simulink model "EPD629_WilliamsJ_AS09_Simulink"  (R2021b)
settings: Solver=VariableStepAuto  StartTime=0.0  StopTime=0.3  MaxStep=0.001  RelTol=1e-3
values from neighbouring files (symbols this model uses):
  b = .001    (= 0.001)    [EPD629_WilliamsJ_AS09.m]
  J = 50e-6    (= 5e-05)    [EPD629_WilliamsJ_AS09.m]
  K = 0.1    [EPD629_WilliamsJ_AS09.m]
  Kb = Kt    (= 0.063)    [EPD629_WilliamsJ_AS09.m]
  Kd5 = NUM{1}(1)    [EPD629_WilliamsJ_AS09.m]
  Ki1 = NUM{1}(2)    [EPD629_WilliamsJ_AS09.m]
  Ki2 = NUM{1}(2)    [EPD629_WilliamsJ_AS09.m]
  Ki3 = NUM{1}(2)    [EPD629_WilliamsJ_AS09.m]
  Ki4 = NUM{1}(2)    [EPD629_WilliamsJ_AS09.m]
  Ki5 = NUM{1}(3)    [EPD629_WilliamsJ_AS09.m]
  Kp1 = NUM{1}(1)    [EPD629_WilliamsJ_AS09.m]
  Kp2 = NUM{1}(1)    [EPD629_WilliamsJ_AS09.m]
  Kp3 = NUM{1}(1)    [EPD629_WilliamsJ_AS09.m]
  Kp4 = NUM{1}(1)    [EPD629_WilliamsJ_AS09.m]
  Kp5 = NUM{1}(2)    [EPD629_WilliamsJ_AS09.m]
  Kt = 0.063    [EPD629_WilliamsJ_AS09.m]
  L = 1e-4    (= 0.0001)    [EPD629_WilliamsJ_AS09.m]
  R = 0.35    [EPD629_WilliamsJ_AS09.m]
  Tau = 0.001    [EPD629_WilliamsJ_AS09.m]
settings Model: Creator=justin  LastModifiedBy=justin

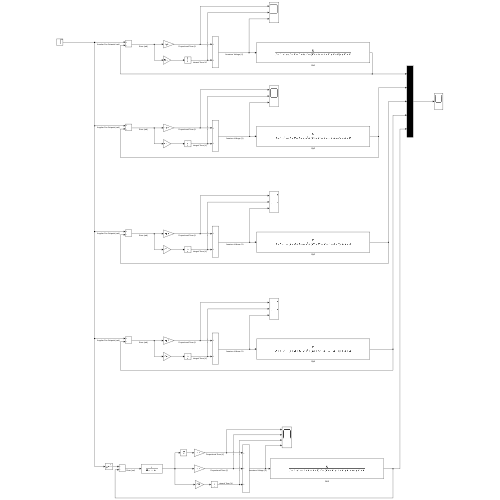
[thumbnail: Simulink's stored preview of the top-level diagram]
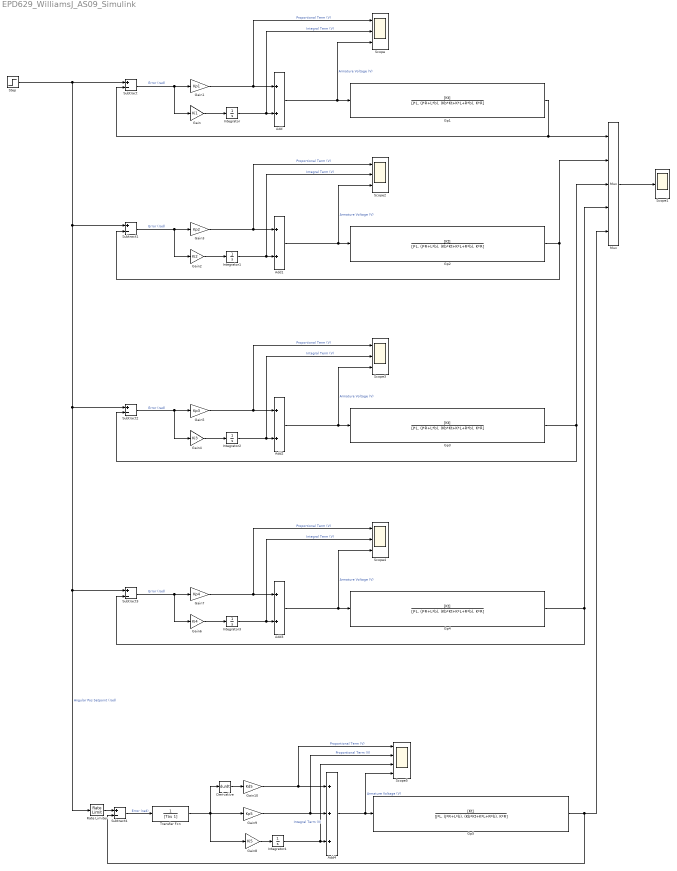
== system EPD629_WilliamsJ_AS09_Simulink ==
  Add{,1..3} (4 alike) : Sum
  Add4 : Sum  Inputs=+++
  Derivative : Derivative
  Gain : Gain  Gain=Ki1
  Gain1 : Gain  Gain=Kp1
  Gain10 : Gain  Gain=Kd5
  Gain2 : Gain  Gain=Ki2
  Gain3 : Gain  Gain=Kp2
  Gain4 : Gain  Gain=Ki3
  Gain5 : Gain  Gain=Kp3
  Gain6 : Gain  Gain=Ki4
  Gain7 : Gain  Gain=Kp4
  Gain8 : Gain  Gain=Ki5
  Gain9 : Gain  Gain=Kp5
  Gp{1..5} (5 alike) : TransferFcn  Numerator=[Kt]  Denominator=[J*L, (J*R+L*b), (Kb*Kt+K*L+R*b), K*R]
  Integrator{,1..4} (5 alike) : Integrator
  Mux : Mux  Inputs=5
  Rate Limiter : RateLimiter  RisingSlewLimit=180  FallingSlewLimit=-180  SampleTimeMode=inherited
  Scope{,2..4} (4 alike) : Scope  NumInputPorts=3
  Scope1 : Scope
  Scope5 : Scope  NumInputPorts=4
  Step : Step  Time=0.1  SampleTime=0
  Subtract{,1..4} (5 alike) : Sum  Inputs=+-
  Transfer Fcn : TransferFcn  Denominator=[Tau 1]
  wires:
  Subtract/1 -> Gain1/1, Gain/1  "Error (rad)"
  Gain/1 -> Integrator/1
  Gain1/1 -> Add/1, Scope/1  "Proportional Term (V)"
  Integrator/1 -> Add/2, Scope/2  "Integral Term (V)"
  Add/1 -> Gp1/1, Scope/3  "Armature Voltage (V)"
  Gp1/1 -> Subtract/2, Mux/1
  Mux/1 -> Scope1/1
  Gp2/1 -> Mux/2, Subtract1/2
  Add1/1 -> Gp2/1, Scope2/3  "Armature Voltage (V)"
  Integrator1/1 -> Scope2/2, Add1/2  "Integral Term (V)"
  Gain3/1 -> Scope2/1, Add1/1  "Proportional Term (V)"
  Gain2/1 -> Integrator1/1
  Subtract1/1 -> Gain2/1, Gain3/1  "Error (rad)"
  Subtract2/1 -> Gain5/1, Gain4/1  "Error (rad)"
  Gain4/1 -> Integrator2/1
  Gain5/1 -> Add2/1, Scope3/1  "Proportional Term (V)"
  Integrator2/1 -> Add2/2, Scope3/2  "Integral Term (V)"
  Add2/1 -> Scope3/3, Gp3/1  "Armature Voltage (V)"
  Gp3/1 -> Mux/3, Subtract2/2
  Step/1 -> Rate Limiter/1, Subtract3/1, Subtract2/1, Subtract1/1, Subtract/1  "Angular Pos Setpoint (rad)"
  Gp4/1 -> Subtract3/2, Mux/4
  Add3/1 -> Gp4/1, Scope4/3  "Armature Voltage (V)"
  Integrator3/1 -> Scope4/2, Add3/2  "Integral Term (V)"
  Gain7/1 -> Scope4/1, Add3/1  "Proportional Term (V)"
  Gain6/1 -> Integrator3/1
  Subtract3/1 -> Gain6/1, Gain7/1  "Error (rad)"
  Subtract4/1 -> Transfer Fcn/1  "Error (rad)"
  Gain8/1 -> Integrator4/1
  Gain9/1 -> Add4/2, Scope5/2  "Proportional Term (V)"
  Integrator4/1 -> Scope5/3, Add4/3  "Integral Term (V)"
  Add4/1 -> Gp5/1, Scope5/4  "Armature Voltage (V)"
  Gp5/1 -> Subtract4/2, Mux/5
  Derivative/1 -> Gain10/1
  Gain10/1 -> Scope5/1, Add4/1  "Proportional Term (V)"
  Rate Limiter/1 -> Subtract4/1
  Transfer Fcn/1 -> Derivative/1, Gain9/1, Gain8/1
